simulink model "mdaqdemo_testanalog"  (R2013a)
settings: Solver=FixedStepDiscrete  SolverMode=SingleTasking  StartTime=0.0  StopTime=inf  FixedStep=0.001  RelTol=1e-3
libraries: microdaq_lib x2
settings Model: SimulationMode=external  ExtModeTrigDuration=10000  Creator=peselnikmg  LastModifiedBy=skibool
settings DataIOCC: SignalLoggingSaveFormat=ModelDataLogs
settings OptimizationCC: OptimizeModelRefInitCode=on  LifeSpan=1
settings DebuggingCC: MultiTaskDSMMsg=warning  MultiTaskCondExecSysMsg=none  StrictBusMsg=None
settings HardwareCC: ProdBitPerLong=40  ProdLargestAtomicInteger=Integer  ProdIntDivRoundTo=Zero  ProdEndianess=LittleEndian  ProdHWDeviceType=Texas Instruments->C6000
settings RTWCC: SystemTargetFile=microdaq.tlc  TemplateMakefile=microdaq.tmf  PostCodeGenCommand=microdaq_postcodegen(buildInfo)  Description=MicroDAQ Real-Time Measurement System  GenerateReport=on  ProcessScript=microdaq_make_rtw_hook  IncludeHyperlinkInReport=on  IncludeERTFirstTime=on
settings CodeAppCC: IgnoreCustomStorageClasses=off
settings STFCustomTargetCC: CodeReplacementLibrary=TI C674x  CombineOutputUpdateFcns=on  ERTCustomFileBanners=on  SupportContinuousTime=off  SupportNonInlinedSFcns=off  MATLABClassNameForMDSCustomization=Simulink.SoftwareTarget.ERTCustomization  SystemTargetFile=microdaq.tlc
settings ERTTargetCC: CodeReplacementLibrary=TI C674x  GenerateSampleERTMain=off  ParMdlRefBuildCompliant=off  CompOptLevelCompliant=off  ConcurrentExecutionCompliant=off  ERTFirstTimeCompliant=off  ModelStepFunctionPrototypeControlCompliant=off  CPPClassGenCompliant=off  ExtMode=on  ExtModeStaticAlloc=on  ExtModeStaticAllocSize=10485760  ExtModeMexArgs=getpref('microdaq','TargetIP') 1 4344  ERTCustomFileTemplate=microdaq_main.tlc

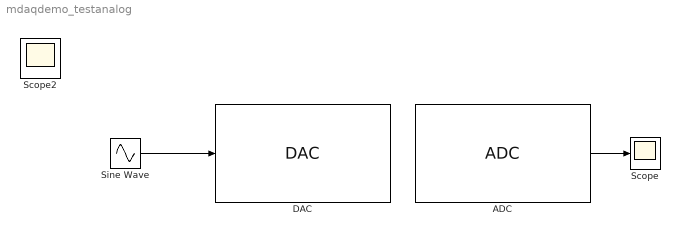
== system mdaqdemo_testanalog ==
  ADC : microdaq_lib/Analog/ADC  Priority=2  pChannel=1  pChannelCount=ones([1 1 ])  pRange=[-10 10]  pMode=0  pAveraging=Off  SampleTime=0.1
      settings: AttributesFormatString=Priority: %<Priority>
  DAC : microdaq_lib/Analog/DAC  Priority=1  pChannel=1  pChannelCount=ones([1 1 ])  pRange=[0 5]  pInitValue=0  pTermValue=0  pUseInitTerm=2  SampleTime=0.1
      settings: AttributesFormatString=Priority: %<Priority>
  Scope : Scope
      settings: YMin=1.25  YMax=3.75
  Sine Wave : Sin  Bias=2.5  SampleTime=0.1
      settings: AttributesFormatString=Sample Time: %<SampleTime>
  Scope2 : Scope
      settings: MaxDataPoints=7500
  wires:
  Sine Wave/1 -> DAC/1
  ADC/1 -> Scope/1
